simulink model "battery_2rc"  (R2022b)
settings: Solver=VariableStepAuto  StartTime=0.0  StopTime=10.0  RelTol=1e-3
undefined symbols (not defined in the file): Battery, I_cc, I_gain, P_gain, R_bleed, T_volt, V_top
libraries: fl_lib x28, nesl_utility x18, simulink x3, batteryecm_lib x3, ee_lib x3, slpidlib x1
(part 2 of 2)

== stateflow chart battery_2rc/Chart ==
  state wait
  state DISCH
    du: MODE = 2;
  state CH
    du: MODE = 1;
  (default) -> wait
  wait -> (junction 14)
  (junction 14) -> (junction 16) [order 1] : [SOC_MAX<0.5]
  (junction 14) -> DISCH [order 2] : [SOC_MAX>=0.5]
  (junction 16) -> (junction 19)
  CH -> DISCH : [SOC_MAX > 0.99 || after(5000,sec)]
  DISCH -> CH : [SOC_min < 0.3]
  (junction 19) -> CH
  data: MODE output; SOC_MAX input; SOC_min input
